simulink model "carPlant_BandoHumanFollower_4"  (R2018b)
settings: Solver=VariableStepAuto  StartTime=0.0  StopTime=inf  RelTol=1e-3
libraries: autolibshared x2, vehdynlibsteering x2
settings Model: Creator=ckreienk  LastModifiedBy=ckreienk

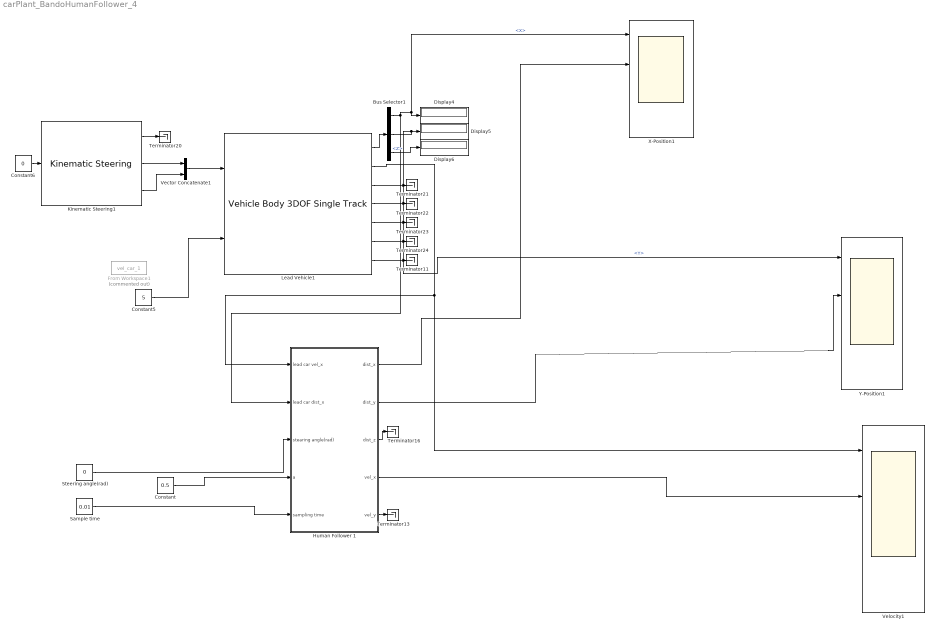
== system carPlant_BandoHumanFollower_4 ==
  Bus Selector1 : BusSelector  OutputSignals=InertFrm.Geom.Disp.X,InertFrm.Geom.Disp.Y,InertFrm.Geom.Disp.Z
  Constant : Constant  Value=0.5
  Constant5 : Constant  Value=5
  Constant6 : Constant  Value=0
  Display4 : Display
  Display5 : Display
  Display6 : Display
  From Workspace1 : FromWorkspace  Commented=on  VariableName=vel_car_1  SampleTime=0.1
  Human Follower 1 : Subsystem
  Kinematic Steering1 : vehdynlibsteering/Kinematic Steering  StrgType=Ackerman  StrgRatioType=Constant  Loc=Front  NrmlFctr=0.01  TrckWdth=1  WhlBase=1.524  Db=0  StrgRng=1.25*pi  StrgAngBpts="[-6.2832   -5.0265   -3.7699   -2.5133   -1.2566         0    1.2566    2.5133    3.7699    5.0265    6.2832]"  StrgRatioTbl=|  StrgRatio=100  StrgArmLngth=0.1  RckCsLngth=0.5  TieRodLngth=0.248  D=0.2  PnnRadius=0.0057  PnnRadiusTbl="[0.0055    0.0055    0.0056    0.0057    0.0058    0.0057    0.0057    0.0057    0.0056    0.0055    0.0055]"  RodLngth=0.1  ParaArmLngth=0.9  aMode=2
      | [13.5000   13.3750   13.2500   13.1250   13.0000   13.0000   13.0000   13.1250   13.2500   13.3750   13.5000
      | ]
      settings: SourceProductName=Vehicle Dynamics Blockset
  Lead Vehicle1 : autolibshared/Vehicle Body 3DOF Single Track  trackMode=Dual  inputMode=External longitudinal velocity  frontSteerMode=on  rearSteerMode=off  windMode=off  muMode=off  extFMode=off  extMMode=off  aMode=2  NF=2  NR=2  m=2000  a=1.4  b=1.6  h=0.35  X_o=4.5  xdot_o=0  CalphaMode=off  sigmaMode=off  d=0  w=[1.4,1.4]  Cy_f=12e3  Cy_r=11e3  sigma_f=.1  sigma_r=.1  alpha_f_brk=[-.1 .1]  Cy_f_data=[-9e3 9e3]  alpha_r_brk=[-.1 .1]  Cy_r_data=[-9e3 9e3]  Y_o=0  ydot_o=0  Izz=4000  psi_o=0  r_o=0  Af=2  Cd=.3  Cl=.1  Cpm=.1  beta_w=[0:0.01:0.3]  Cs=[0:0.03:0.9]  Cym=[0:0.01:0.3]  Pabs=101325  Tair=273  g=9.81  mu=1  xdot_tol=.01  Fznom=5000  Fxtire_sat=7e4  Fytire_sat=7e4  longOff=0  latOff=0  vertOff=0
      settings: SourceProductName=Powertrain Blockset  SourceProductBaseCode=PW
  Sample time : Constant  Value=0.01
  Steering angle(rad) : Constant  Value=0
  Terminator{11,13,16,20..24} (8 alike) : Terminator
  Vector Concatenate1 : Concatenate
  Velocity1 : Scope  NumInputPorts=4
  X-Position1 : Scope  NumInputPorts=4
  Y-Position1 : Scope  NumInputPorts=4
  wires:
  Human Follower 1/2(dist_y) -> Y-Position1/2
  Vector Concatenate1/1 -> Lead Vehicle1/1
  Lead Vehicle1/7 -> Terminator11/1
  Human Follower 1/1(dist_x) -> X-Position1/2
  Sample time/1 -> Human Follower 1/5(sampling time)
  Lead Vehicle1/6 -> Terminator24/1
  Bus Selector1/1 -> Display4/1, X-Position1/1, Human Follower 1/2(lead car dist_x)  "<X>"
  Kinematic Steering1/2 -> Vector Concatenate1/1
  Lead Vehicle1/3 -> Terminator21/1
  Lead Vehicle1/4 -> Terminator22/1
  Human Follower 1/3(dist_z) -> Terminator16/1
  Lead Vehicle1/2 -> Velocity1/1, Human Follower 1/1(lead car vel_x)
  Constant6/1 -> Kinematic Steering1/1
  Constant5/1 -> Lead Vehicle1/2
  Lead Vehicle1/1 -> Bus Selector1/1
  Bus Selector1/2 -> Display5/1, Y-Position1/1  "<Y>"
  Kinematic Steering1/1 -> Terminator20/1
  Kinematic Steering1/3 -> Vector Concatenate1/2
  Bus Selector1/3 -> Display6/1  "<Z>"
  Human Follower 1/5(vel_y) -> Terminator13/1
  Lead Vehicle1/5 -> Terminator23/1
  Steering angle(rad)/1 -> Human Follower 1/3(stearing angle(rad))
  Constant/1 -> Human Follower 1/4(a)
  Human Follower 1/4(vel_x) -> Velocity1/2

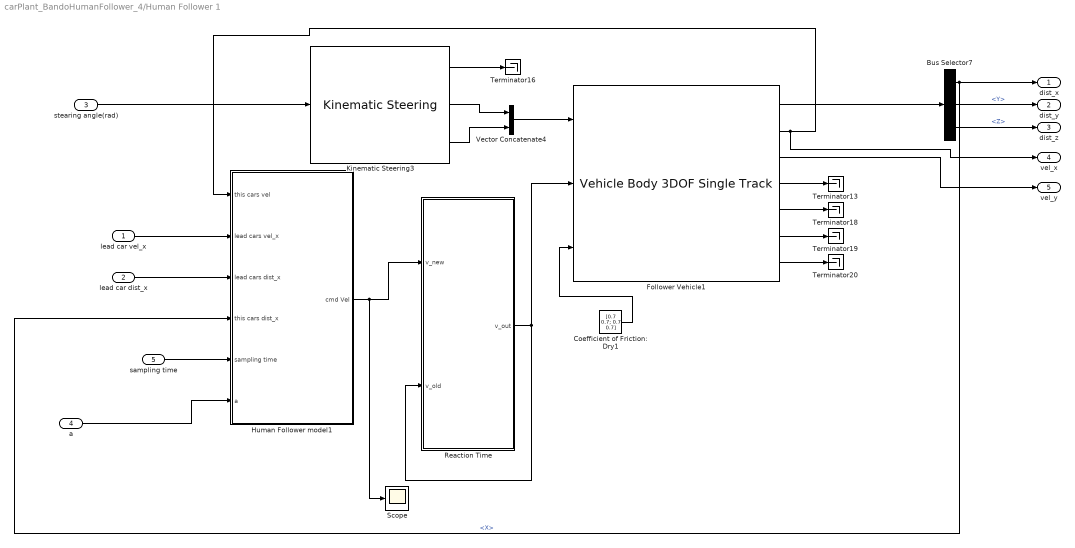
== system carPlant_BandoHumanFollower_4/Human Follower 1 ==
  lead car vel_x : Inport
  lead car dist_x : Inport  Port=2
  stearing angle(rad) : Inport  Port=3
  a : Inport  Port=4
  sampling time : Inport  Port=5
  Bus Selector7 : BusSelector  OutputSignals=InertFrm.Cg.Disp.X,InertFrm.Cg.Disp.Y,InertFrm.Cg.Disp.Z
  Coefficient of Friction: Dry1 : Constant  Value=[0.7 0.7; 0.7 0.7]
  Follower Vehicle1 : autolibshared/Vehicle Body 3DOF Single Track  trackMode=Dual  inputMode=External longitudinal velocity  frontSteerMode=on  rearSteerMode=off  windMode=off  muMode=on  extFMode=off  extMMode=off  aMode=2  NF=2  NR=2  m=2000  a=1.4  b=1.6  h=0.35  X_o=0  xdot_o=0  CalphaMode=off  sigmaMode=on  d=0  w=[1.4,1.4]  Cy_f=12e3  Cy_r=11e3  sigma_f=.1  sigma_r=.1  alpha_f_brk=[-.1 .1]  Cy_f_data=[-9e3 9e3]  alpha_r_brk=[-.1 .1]  Cy_r_data=[-9e3 9e3]  Y_o=0  ydot_o=0  Izz=4000  psi_o=0  r_o=0  Af=2  Cd=.3  Cl=.1  Cpm=.1  beta_w=[0:0.01:0.3]  Cs=[0:0.03:0.9]  Cym=[0:0.01:0.3]  Pabs=101325  Tair=273  g=9.81  mu=1  xdot_tol=.01  Fznom=5000  Fxtire_sat=7e4  Fytire_sat=7e4  longOff=0  latOff=0  vertOff=0
      settings: SourceProductName=Powertrain Blockset  SourceProductBaseCode=PW
  Human Follower model1 : Subsystem
  Kinematic Steering3 : vehdynlibsteering/Kinematic Steering  StrgType=Ackerman  StrgRatioType=Constant  Loc=Front  NrmlFctr=0.01  TrckWdth=1  WhlBase=1.524  Db=0  StrgRng=1.25*pi  StrgAngBpts="[-6.2832   -5.0265   -3.7699   -2.5133   -1.2566         0    1.2566    2.5133    3.7699    5.0265    6.2832]"  StrgRatioTbl=|  StrgRatio=100  StrgArmLngth=0.1  RckCsLngth=0.5  TieRodLngth=0.248  D=0.2  PnnRadius=0.0057  PnnRadiusTbl="[0.0055    0.0055    0.0056    0.0057    0.0058    0.0057    0.0057    0.0057    0.0056    0.0055    0.0055]"  RodLngth=0.1  ParaArmLngth=0.9  aMode=2
      | [13.5000   13.3750   13.2500   13.1250   13.0000   13.0000   13.0000   13.1250   13.2500   13.3750   13.5000
      | ]
      settings: SourceProductName=Vehicle Dynamics Blockset
  Reaction Time : Subsystem
  Scope : Scope
  Terminator{13,16,18..20} (5 alike) : Terminator
  Vector Concatenate4 : Concatenate
  dist_x : Outport
  dist_y : Outport  Port=2
  dist_z : Outport  Port=3
  vel_x : Outport  Port=4
  vel_y : Outport  Port=5
  wires:
  Bus Selector7/3 -> dist_z/1  "<Z>"
  Follower Vehicle1/5 -> Terminator18/1
  Follower Vehicle1/6 -> Terminator19/1
  Bus Selector7/1 -> Human Follower model1/4(this cars dist_x), dist_x/1  "<X>"
  Follower Vehicle1/4 -> Terminator13/1
  Follower Vehicle1/3 -> vel_y/1
  lead car vel_x/1 -> Human Follower model1/2(lead cars vel_x)
  Follower Vehicle1/7 -> Terminator20/1
  Vector Concatenate4/1 -> Follower Vehicle1/1
  Follower Vehicle1/1 -> Bus Selector7/1
  Kinematic Steering3/1 -> Terminator16/1
  Bus Selector7/2 -> dist_y/1  "<Y>"
  Kinematic Steering3/2 -> Vector Concatenate4/1
  stearing angle(rad)/1 -> Kinematic Steering3/1
  Kinematic Steering3/3 -> Vector Concatenate4/2
  Follower Vehicle1/2 -> Human Follower model1/1(this cars vel), vel_x/1
  Coefficient of Friction: Dry1/1 -> Follower Vehicle1/3
  a/1 -> Human Follower model1/6(a)
  Reaction Time/1(v_out) -> Follower Vehicle1/2, Reaction Time/2(v_old)
  Human Follower model1/1(cmd Vel) -> Scope/1, Reaction Time/1(v_new)
  lead car dist_x/1 -> Human Follower model1/3(lead cars dist_x)
  sampling time/1 -> Human Follower model1/5(sampling time)

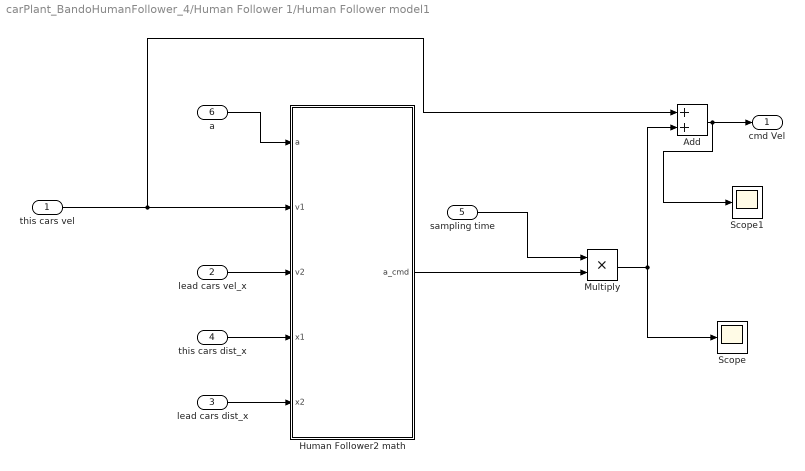
== system carPlant_BandoHumanFollower_4/Human Follower 1/Human Follower model1 ==
  this cars vel : Inport
  lead cars vel_x : Inport  Port=2
  lead cars dist_x : Inport  Port=3
  this cars dist_x : Inport  Port=4
  sampling time : Inport  Port=5
  a : Inport  Port=6
  Add : Sum
  Human Follower2 math : Subsystem
  Multiply : Product
  Scope : Scope
  Scope1 : Scope
  cmd Vel : Outport
  wires:
  sampling time/1 -> Multiply/1
  Multiply/1 -> Scope/1, Add/2
  Human Follower2 math/1(a_cmd) -> Multiply/2
  this cars vel/1 -> Human Follower2 math/2(v1), Add/1
  Add/1 -> Scope1/1, cmd Vel/1
  a/1 -> Human Follower2 math/1(a)
  lead cars dist_x/1 -> Human Follower2 math/5(x2)
  lead cars vel_x/1 -> Human Follower2 math/3(v2)
  this cars dist_x/1 -> Human Follower2 math/4(x1)

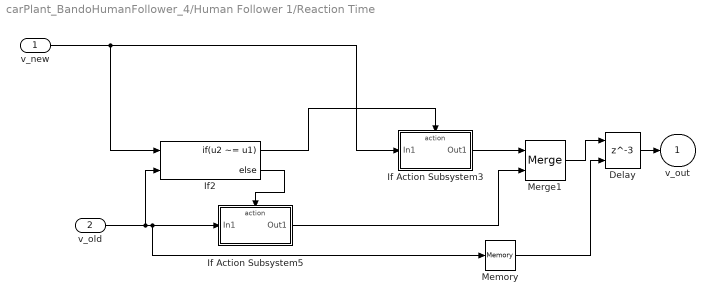
== system carPlant_BandoHumanFollower_4/Human Follower 1/Reaction Time ==
  v_new : Inport
  v_old : Inport  Port=2
  Delay : Delay  DelayLength=3  InitialConditionSource=Input port
      settings: InputPortMap=u0,p4
  If Action Subsystem3 : Subsystem  TreatAsAtomicUnit=on
  If Action Subsystem5 : Subsystem  TreatAsAtomicUnit=on
  If2 : If  NumInputs=2  IfExpression=u2 ~= u1
  Memory : Memory
  Merge1 : Merge
  v_out : Outport
  wires:
  v_old/1 -> If2/2, Memory/1, If Action Subsystem5/1(In1)
  If Action Subsystem5/1(Out1) -> Merge1/2
  If2/1 -> If Action Subsystem3/Action
  If2/2 -> If Action Subsystem5/Action
  If Action Subsystem3/1(Out1) -> Merge1/1
  v_new/1 -> If2/1, If Action Subsystem3/1(In1)
  Merge1/1 -> Delay/1
  Delay/1 -> v_out/1
  Memory/1 -> Delay/2

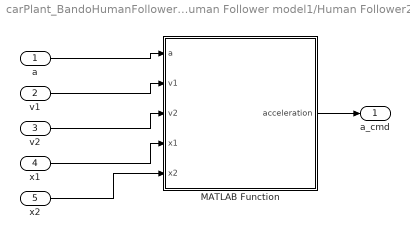
== system carPlant_BandoHumanFollower_4/Human Follower 1/Human Follower model1/Human Follower2 math ==
  a : Inport
  v1 : Inport  Port=2
  v2 : Inport  Port=3
  x1 : Inport  Port=4
  x2 : Inport  Port=5
  MATLAB Function : MATLAB Function  TreatAsAtomicUnit=on
  a_cmd : Outport
  wires:
  v1/1 -> MATLAB Function/2(v1)
  a/1 -> MATLAB Function/1(a)
  v2/1 -> MATLAB Function/3(v2)
  MATLAB Function/1(acceleration) -> a_cmd/1
  x1/1 -> MATLAB Function/4(x1)
  x2/1 -> MATLAB Function/5(x2)

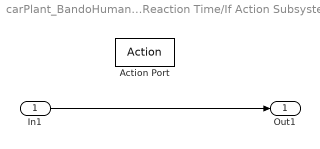
== system carPlant_BandoHumanFollower_4/Human Follower 1/Reaction Time/If Action Subsystem3 ==
  In1 : Inport
  Action Port : ActionPort  ActionType=then
  Out1 : Outport
  wires:
  In1/1 -> Out1/1

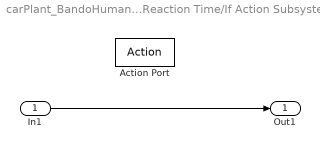
== system carPlant_BandoHumanFollower_4/Human Follower 1/Reaction Time/If Action Subsystem5 ==
  In1 : Inport
  Action Port : ActionPort  ActionType=else
  Out1 : Outport
  wires:
  In1/1 -> Out1/1

== matlab function carPlant_BandoHumanFollower_4/Human Follower 1/Human Follower model1/Human Follower2 math/MATLAB Function ==
  data: a input; v1 input; v2 input; x1 input; acceleration output; x2 input
function acceleration = fcn(a, v1, v2, x1, x2)


if x2 == 0
    x2 = 0.1;
end

acceleration = a*(v2 - v1) / (x2 - x1);
